simulink model "lab3"  (R2014b)
settings: Solver=VariableStepAuto  StartTime=0.0  StopTime=10.0  RelTol=1e-3
values from neighbouring files (symbols this model uses):
  Ts = 0.5    [main.m]
libraries: simulink x1, truetime x1
settings Model: Creator=peterfj  LastModifiedBy=peterfj
settings DataIOCC: SaveFormat=Dataset
settings OptimizationCC: UseDivisionForNetSlopeComputation=off  SimCompilerOptimization=off
settings DebuggingCC: SolverPrmCheckMsg=none  FrameProcessingCompatibilityMsg=error  AllowSymbolicDim=off
settings HardwareCC: ProdBitPerPointer=64  ProdLargestAtomicFloat=Float  ProdIntDivRoundTo=Zero  ProdEndianess=LittleEndian  ProdWordSize=64  ProdHWDeviceType=Intel->x86-64 (Windows64)
settings RTWCC: RTWCompilerOptimization=off
settings GRTTargetCC: GeneratePreprocessorConditionals=Use local settings
settings ConfigComp: CovMetricSettings=dw  CovHtmlReporting=on  CovSaveCumulativeToWorkspaceVar=on  CovSaveSingleToWorkspaceVar=on  CovExternalEMLEnable=off

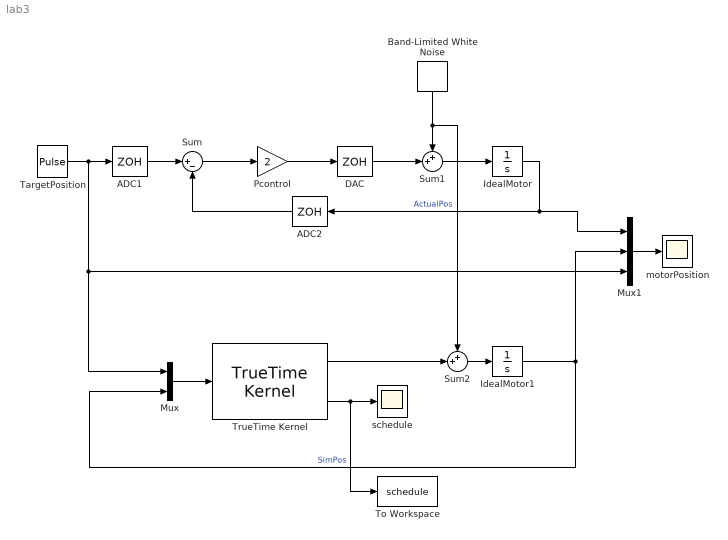
== system lab3 ==
  ADC1 : ZeroOrderHold  SampleTime=Ts
  ADC2 : ZeroOrderHold  SampleTime=Ts
  Band-Limited White Noise : simulink/Sources/Band-Limited White Noise  Cov=[0.1]  Ts=Ts  seed=[23341]
  DAC : ZeroOrderHold  SampleTime=Ts
  IdealMotor : Integrator
  IdealMotor1 : Integrator
  Mux : Mux  Inputs=2
  Mux1 : Mux  Inputs=3
  Pcontrol : Gain  Gain=2
  Sum : Sum  Inputs=|+-
  Sum1 : Sum  Inputs=++|
  Sum2 : Sum  Inputs=++|
  TargetPosition : DiscretePulseGenerator  PulseType=Time based  Period=5  PulseWidth=50
  To Workspace : ToWorkspace  VariableName=schedule  SaveFormat=Timeseries  SampleTime=-1
  TrueTime Kernel : truetime/TrueTime Kernel  sfun=simple_init  args=Ts  ninputsoutputs=[2 1]  ntriggers=0  trigtype=falling  nwnodenbr=[]  clockoffsetdrift=[0 0]  schedoutput=on  battery=off  poweroutput=off
  motorPosition : Scope
      settings: ShowLegends=on  YMin=-0.71542  YMax=1.10202
  schedule : Scope
      settings: YMin=-0.71542  YMax=1.10202
  wires:
  TargetPosition/1 -> Mux/1, Mux1/3, ADC1/1
  ADC1/1 -> Sum/1
  Sum/1 -> Pcontrol/1
  Pcontrol/1 -> DAC/1
  DAC/1 -> Sum1/2
  Band-Limited White Noise/1 -> Sum2/1, Sum1/1
  Sum1/1 -> IdealMotor/1
  IdealMotor/1 -> ADC2/1, Mux1/1  "ActualPos"
  ADC2/1 -> Sum/2
  Mux/1 -> TrueTime Kernel/1
  Mux1/1 -> motorPosition/1
  Sum2/1 -> IdealMotor1/1
  TrueTime Kernel/1 -> Sum2/2
  IdealMotor1/1 -> Mux1/2, Mux/2  "SimPos"
  TrueTime Kernel/2 -> To Workspace/1, schedule/1
